simulink model "firmware_requirements_doc_model"  (R2021b)
settings: Solver=VariableStepAuto  StartTime=0.0  StopTime=10.0  RelTol=1e-3
settings Model: Creator=matas  LastModifiedBy=matas

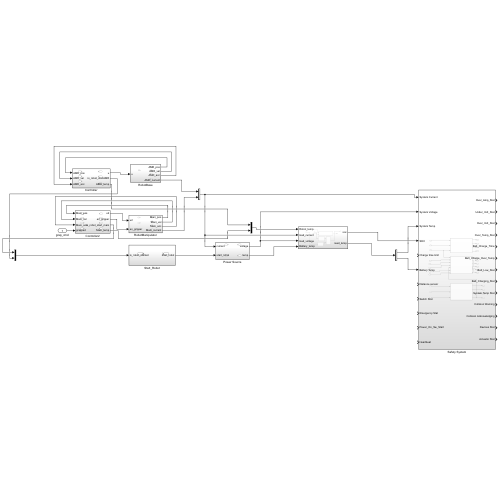
[thumbnail: Simulink's stored preview of the top-level diagram]
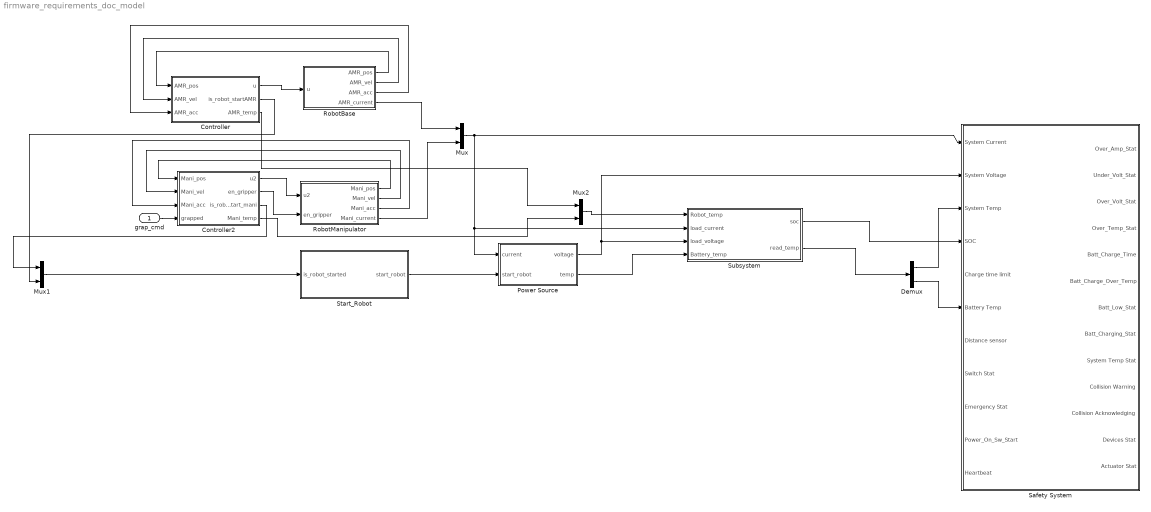
== system firmware_requirements_doc_model ==
  grap_cmd : Inport
  Controller : Subsystem
  Controller2 : Subsystem
  Demux : Demux  Outputs=2
  Mux : Mux  Inputs=2
  Mux1 : Mux  Inputs=2
  Mux2 : Mux  Inputs=2
  Power Source : Subsystem
  RobotBase : Subsystem
  RobotManipulator : Subsystem
  Safety System : Subsystem
  Start_Robot : Subsystem
  Subsystem : Subsystem
  wires:
  Controller2/2(en_gripper) -> RobotManipulator/2(en_gripper)
  Controller2/1(u2) -> RobotManipulator/1(u2)
  Controller/1(u) -> RobotBase/1(u)
  RobotBase/1(AMR_pos) -> Controller/1(AMR_pos)
  RobotBase/2(AMR_vel) -> Controller/2(AMR_vel)
  RobotBase/3(AMR_acc) -> Controller/3(AMR_acc)
  RobotManipulator/1(Mani_pos) -> Controller2/1(Mani_pos)
  RobotManipulator/2(Mani_vel) -> Controller2/2(Mani_vel)
  RobotManipulator/3(Mani_acc) -> Controller2/3(Mani_acc)
  grap_cmd/1 -> Controller2/4(grapped)
  Mux/1 -> Power Source/1(current), Subsystem/2(load_current), Safety System/1(System Current)
  Power Source/1(voltage) -> Subsystem/3(load_voltage), Safety System/2(System Voltage)
  RobotManipulator/4(Mani_current) -> Mux/2
  RobotBase/4(AMR_current) -> Mux/1
  Start_Robot/1(start_robot) -> Power Source/2(start_robot)
  Mux1/1 -> Start_Robot/1(is_robot_started)
  Controller/2(is_robot_startAMR) -> Mux1/2
  Controller2/3(is_robot_start_mani) -> Mux1/1
  Controller/3(AMR_temp) -> Mux2/1
  Controller2/4(Mani_temp) -> Mux2/2
  Demux/1 -> Safety System/3(System Temp)
  Demux/2 -> Safety System/6(Battery Temp)
  Mux2/1 -> Subsystem/1(Robot_temp)
  Power Source/2(temp) -> Subsystem/4(Battery_temp)
  Subsystem/1(soc) -> Safety System/4(SOC)
  Subsystem/2(read_temp) -> Demux/1

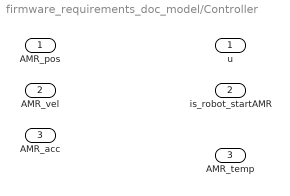
== system firmware_requirements_doc_model/Controller ==
  AMR_pos : Inport
  AMR_vel : Inport  Port=2
  AMR_acc : Inport  Port=3
  u : Outport
  is_robot_startAMR : Outport  Port=2
  AMR_temp : Outport  Port=3

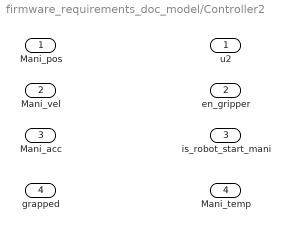
== system firmware_requirements_doc_model/Controller2 ==
  Mani_pos : Inport
  Mani_vel : Inport  Port=2
  Mani_acc : Inport  Port=3
  grapped : Inport  Port=4
  u2 : Outport
  en_gripper : Outport  Port=2
  is_robot_start_mani : Outport  Port=3
  Mani_temp : Outport  Port=4

== system firmware_requirements_doc_model/Power Source ==
  current : Inport
  start_robot : Inport  Port=2
  voltage : Outport
  temp : Outport  Port=2

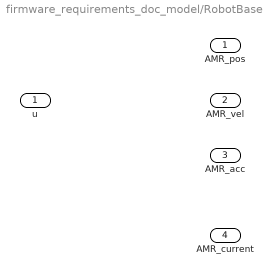
== system firmware_requirements_doc_model/RobotBase ==
  u : Inport
  AMR_pos : Outport
  AMR_vel : Outport  Port=2
  AMR_acc : Outport  Port=3
  AMR_current : Outport  Port=4

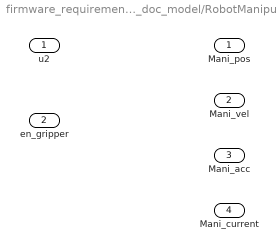
== system firmware_requirements_doc_model/RobotManipulator ==
  u2 : Inport
  en_gripper : Inport  Port=2
  Mani_pos : Outport
  Mani_vel : Outport  Port=2
  Mani_acc : Outport  Port=3
  Mani_current : Outport  Port=4

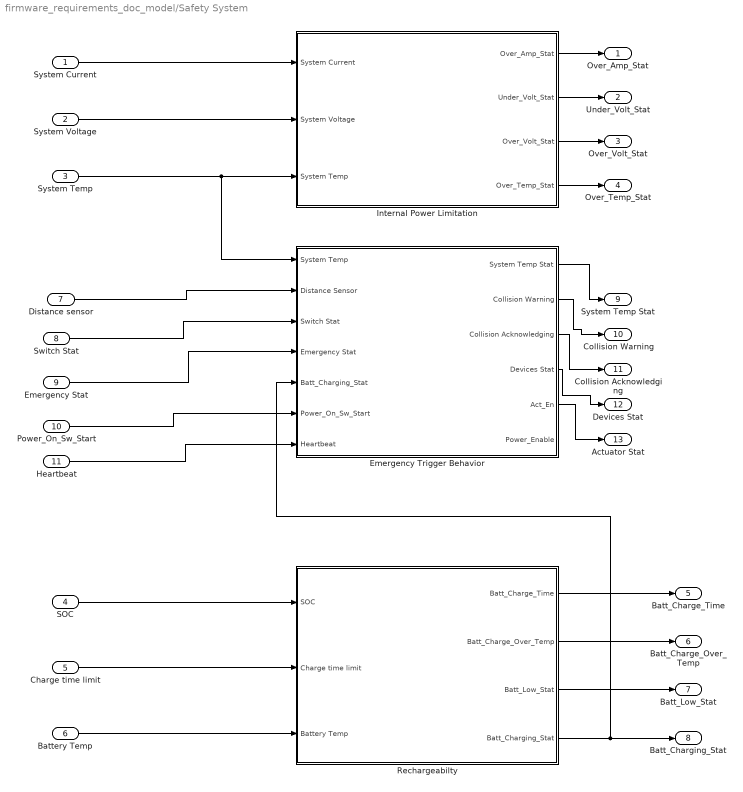
== system firmware_requirements_doc_model/Safety System ==
  System Current : Inport
  System Voltage : Inport  Port=2
  System Temp : Inport  Port=3
  SOC : Inport  Port=4
  Charge time limit : Inport  Port=5
  Battery Temp : Inport  Port=6
  Distance sensor : Inport  Port=7
  Switch Stat : Inport  Port=8
  Emergency Stat : Inport  Port=9
  Power_On_Sw_Start : Inport  Port=10
  Heartbeat : Inport  Port=11
  Emergency Trigger Behavior : Subsystem
  Internal Power Limitation : Subsystem
  Rechargeabilty : Subsystem
  Over_Amp_Stat : Outport
  Under_Volt_Stat : Outport  Port=2
  Over_Volt_Stat : Outport  Port=3
  Over_Temp_Stat : Outport  Port=4
  Batt_Charge_Time : Outport  Port=5
  Batt_Charge_Over_Temp : Outport  Port=6
  Batt_Low_Stat : Outport  Port=7
  Batt_Charging_Stat : Outport  Port=8
  System Temp Stat : Outport  Port=9
  Collision Warning : Outport  Port=10
  Collision Acknowledging : Outport  Port=11
  Devices Stat : Outport  Port=12
  Actuator Stat : Outport  Port=13
  wires:
  System Temp/1 -> Internal Power Limitation/3(System Temp), Emergency Trigger Behavior/1(System Temp)
  System Voltage/1 -> Internal Power Limitation/2(System Voltage)
  Rechargeabilty/1(Batt_Charge_Time) -> Batt_Charge_Time/1
  Rechargeabilty/2(Batt_Charge_Over_Temp) -> Batt_Charge_Over_Temp/1
  Rechargeabilty/3(Batt_Low_Stat) -> Batt_Low_Stat/1
  System Current/1 -> Internal Power Limitation/1(System Current)
  Internal Power Limitation/4(Over_Temp_Stat) -> Over_Temp_Stat/1
  Rechargeabilty/4(Batt_Charging_Stat) -> Emergency Trigger Behavior/5(Batt_Charging_Stat), Batt_Charging_Stat/1
  Internal Power Limitation/1(Over_Amp_Stat) -> Over_Amp_Stat/1
  Internal Power Limitation/2(Under_Volt_Stat) -> Under_Volt_Stat/1
  Internal Power Limitation/3(Over_Volt_Stat) -> Over_Volt_Stat/1
  SOC/1 -> Rechargeabilty/1(SOC)
  Battery Temp/1 -> Rechargeabilty/3(Battery Temp)
  Charge time limit/1 -> Rechargeabilty/2(Charge time limit)
  Distance sensor/1 -> Emergency Trigger Behavior/2(Distance Sensor)
  Emergency Trigger Behavior/4(Devices Stat) -> Devices Stat/1
  Emergency Trigger Behavior/3(Collision Acknowledging) -> Collision Acknowledging/1
  Emergency Trigger Behavior/1(System Temp Stat) -> System Temp Stat/1
  Emergency Trigger Behavior/5(Act_En) -> Actuator Stat/1
  Emergency Trigger Behavior/2(Collision Warning) -> Collision Warning/1
  Switch Stat/1 -> Emergency Trigger Behavior/3(Switch Stat)
  Emergency Stat/1 -> Emergency Trigger Behavior/4(Emergency Stat)
  Power_On_Sw_Start/1 -> Emergency Trigger Behavior/6(Power_On_Sw_Start)
  Heartbeat/1 -> Emergency Trigger Behavior/7(Heartbeat)

== system firmware_requirements_doc_model/Start_Robot ==
  is_robot_started : Inport
  start_robot : Outport

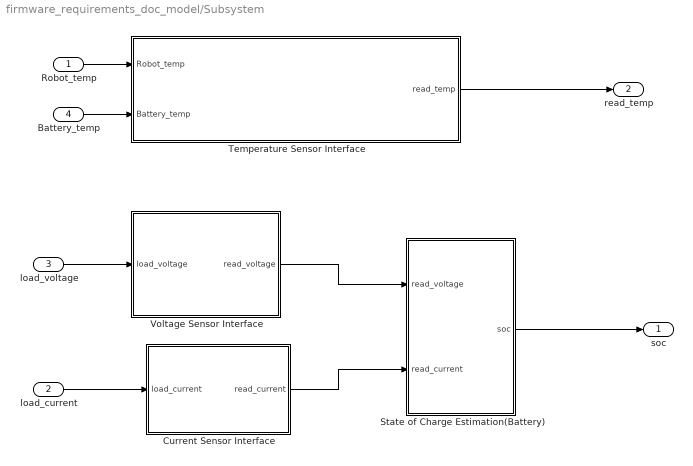
== system firmware_requirements_doc_model/Subsystem ==
  Robot_temp : Inport
  load_current : Inport  Port=2
  load_voltage : Inport  Port=3
  Battery_temp : Inport  Port=4
  Current Sensor Interface : Subsystem
  State of Charge Estimation(Battery) : Subsystem
  Temperature Sensor Interface : Subsystem
  Voltage Sensor Interface : Subsystem
  soc : Outport
  read_temp : Outport  Port=2
  wires:
  Temperature Sensor Interface/1(read_temp) -> read_temp/1
  State of Charge Estimation(Battery)/1(soc) -> soc/1
  Current Sensor Interface/1(read_current) -> State of Charge Estimation(Battery)/2(read_current)
  load_voltage/1 -> Voltage Sensor Interface/1(load_voltage)
  Voltage Sensor Interface/1(read_voltage) -> State of Charge Estimation(Battery)/1(read_voltage)
  Robot_temp/1 -> Temperature Sensor Interface/1(Robot_temp)
  load_current/1 -> Current Sensor Interface/1(load_current)
  Battery_temp/1 -> Temperature Sensor Interface/2(Battery_temp)

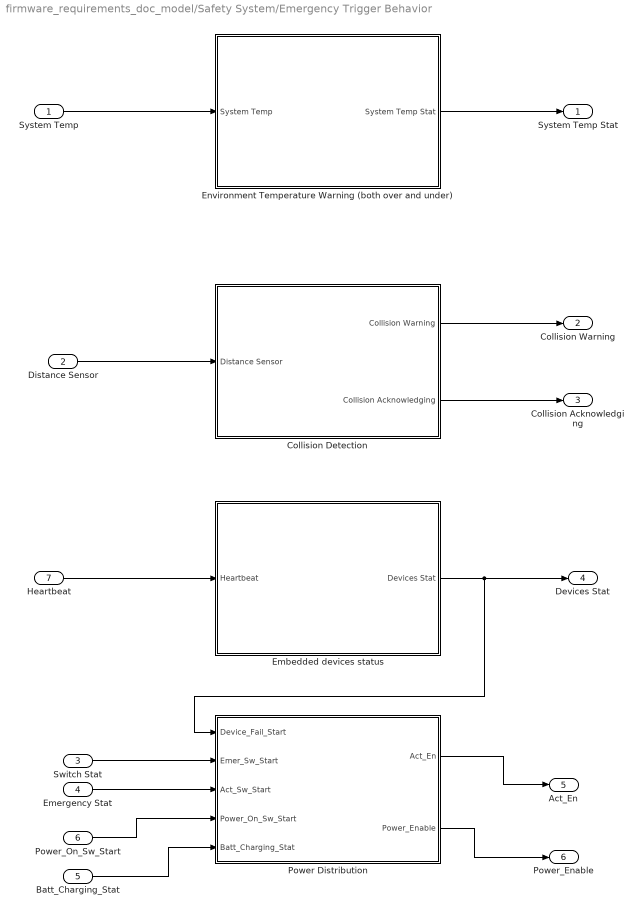
== system firmware_requirements_doc_model/Safety System/Emergency Trigger Behavior ==
  System Temp : Inport
  Distance Sensor : Inport  Port=2
  Switch Stat : Inport  Port=3
  Emergency Stat : Inport  Port=4
  Batt_Charging_Stat : Inport  Port=5
  Power_On_Sw_Start : Inport  Port=6
  Heartbeat : Inport  Port=7
  Collision Detection : Subsystem
  Embedded devices status : Subsystem
  Environment Temperature Warning (both over and under) : Subsystem
  Power Distribution : Subsystem
  System Temp Stat : Outport
  Collision Warning : Outport  Port=2
  Collision Acknowledging : Outport  Port=3
  Devices Stat : Outport  Port=4
  Act_En : Outport  Port=5
  Power_Enable : Outport  Port=6
  wires:
  System Temp/1 -> Environment Temperature Warning (both over and under)/1(System Temp)
  Environment Temperature Warning (both over and under)/1(System Temp Stat) -> System Temp Stat/1
  Distance Sensor/1 -> Collision Detection/1(Distance Sensor)
  Collision Detection/1(Collision Warning) -> Collision Warning/1
  Collision Detection/2(Collision Acknowledging) -> Collision Acknowledging/1
  Power Distribution/1(Act_En) -> Act_En/1
  Switch Stat/1 -> Power Distribution/2(Emer_Sw_Start)
  Emergency Stat/1 -> Power Distribution/3(Act_Sw_Start)
  Batt_Charging_Stat/1 -> Power Distribution/5(Batt_Charging_Stat)
  Power_On_Sw_Start/1 -> Power Distribution/4(Power_On_Sw_Start)
  Embedded devices status/1(Devices Stat) -> Power Distribution/1(Device_Fail_Start), Devices Stat/1
  Power Distribution/2(Power_Enable) -> Power_Enable/1
  Heartbeat/1 -> Embedded devices status/1(Heartbeat)

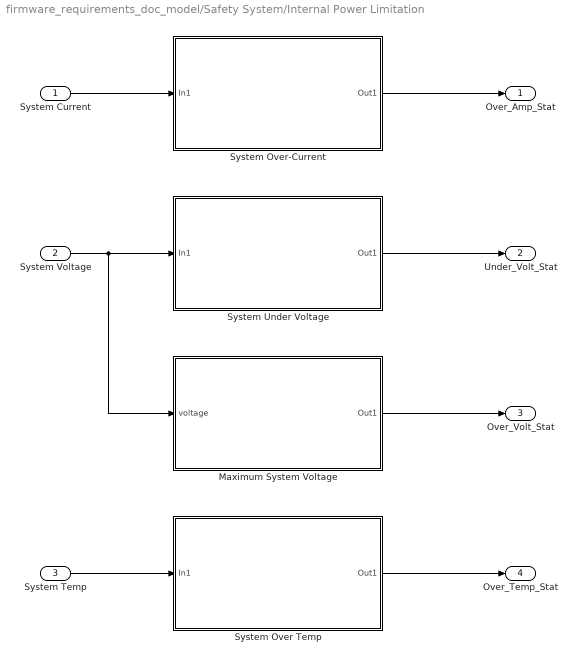
== system firmware_requirements_doc_model/Safety System/Internal Power Limitation ==
  System Current : Inport
  System Voltage : Inport  Port=2
  System Temp : Inport  Port=3
  Maximum System Voltage : Subsystem
  System Over Temp : Subsystem
  System Over-Current : Subsystem
  System Under Voltage : Subsystem
  Over_Amp_Stat : Outport
  Under_Volt_Stat : Outport  Port=2
  Over_Volt_Stat : Outport  Port=3
  Over_Temp_Stat : Outport  Port=4
  wires:
  System Current/1 -> System Over-Current/1(In1)
  System Temp/1 -> System Over Temp/1(In1)
  System Voltage/1 -> Maximum System Voltage/1(voltage), System Under Voltage/1(In1)
  System Over-Current/1(Out1) -> Over_Amp_Stat/1
  System Under Voltage/1(Out1) -> Under_Volt_Stat/1
  Maximum System Voltage/1(Out1) -> Over_Volt_Stat/1
  System Over Temp/1(Out1) -> Over_Temp_Stat/1

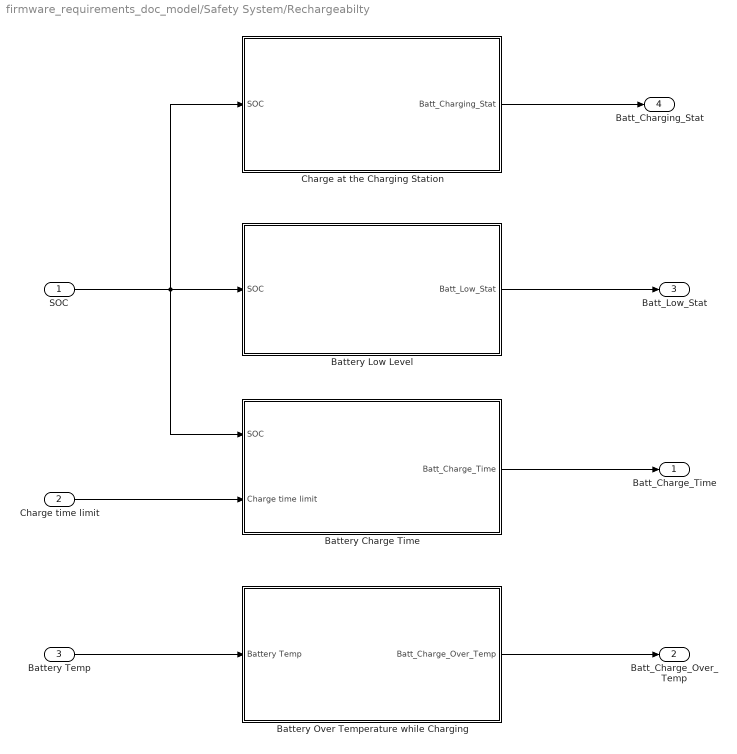
== system firmware_requirements_doc_model/Safety System/Rechargeabilty ==
  SOC : Inport
  Charge time limit : Inport  Port=2
  Battery Temp : Inport  Port=3
  Battery Charge Time : Subsystem
  "Battery Low Level " : Subsystem
  Battery Over Temperature while Charging : Subsystem
  Charge at the Charging Station : Subsystem
  Batt_Charge_Time : Outport
  Batt_Charge_Over_Temp : Outport  Port=2
  Batt_Low_Stat : Outport  Port=3
  Batt_Charging_Stat : Outport  Port=4
  wires:
  Battery Charge Time/1(Batt_Charge_Time) -> Batt_Charge_Time/1
  Charge time limit/1 -> Battery Charge Time/2(Charge time limit)
  Battery Temp/1 -> Battery Over Temperature while Charging/1(Battery Temp)
  Battery Over Temperature while Charging/1(Batt_Charge_Over_Temp) -> Batt_Charge_Over_Temp/1
  "Battery Low Level "/1(Batt_Low_Stat) -> Batt_Low_Stat/1
  SOC/1 -> Battery Charge Time/1(SOC), Charge at the Charging Station/1(SOC), "Battery Low Level "/1(SOC)
  Charge at the Charging Station/1(Batt_Charging_Stat) -> Batt_Charging_Stat/1

== system firmware_requirements_doc_model/Subsystem/Current Sensor Interface ==
  load_current : Inport
  read_current : Outport

== system firmware_requirements_doc_model/Subsystem/State of Charge Estimation(Battery) ==
  read_voltage : Inport
  read_current : Inport  Port=2
  soc : Outport

== system firmware_requirements_doc_model/Subsystem/Temperature Sensor Interface ==
  Robot_temp : Inport
  Battery_temp : Inport  Port=2
  read_temp : Outport

== system firmware_requirements_doc_model/Subsystem/Voltage Sensor Interface ==
  load_voltage : Inport
  read_voltage : Outport

== system firmware_requirements_doc_model/Safety System/Emergency Trigger Behavior/Collision Detection ==
  Distance Sensor : Inport
  Collision Warning : Outport
  Collision Acknowledging : Outport  Port=2

== system firmware_requirements_doc_model/Safety System/Emergency Trigger Behavior/Embedded devices status ==
  Heartbeat : Inport
  Devices Stat : Outport
  wires:
  Heartbeat/1 -> Devices Stat/1

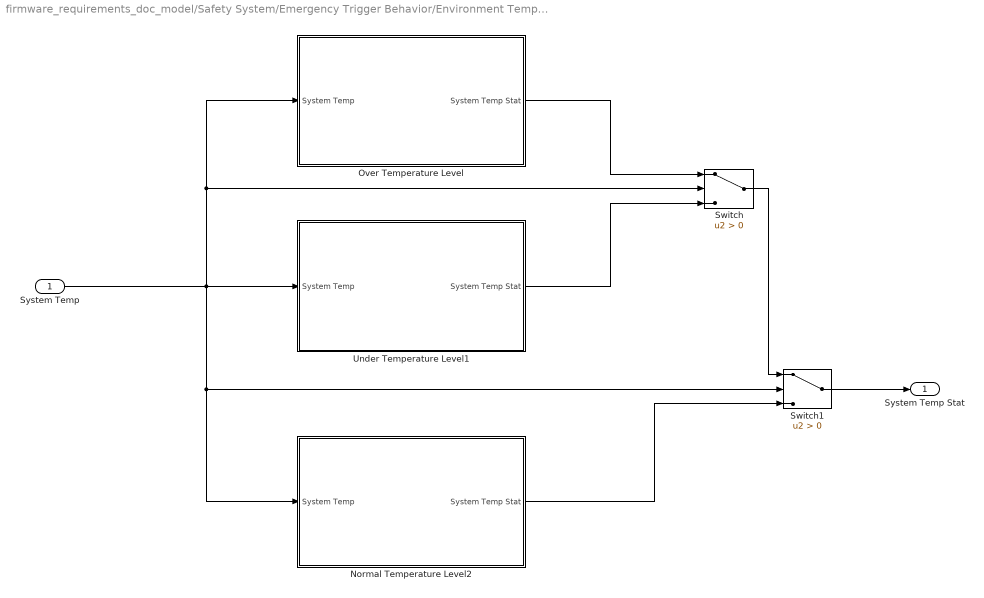
== system firmware_requirements_doc_model/Safety System/Emergency Trigger Behavior/Environment Temperature Warning (both over and under) ==
  System Temp : Inport
  Normal Temperature Level2 : Subsystem
  Over Temperature Level : Subsystem
  Switch : Switch  Criteria=u2 > Threshold
  Switch1 : Switch  Criteria=u2 > Threshold
  Under Temperature Level1 : Subsystem
  System Temp Stat : Outport
  wires:
  System Temp/1 -> Normal Temperature Level2/1(System Temp), Switch1/2, Under Temperature Level1/1(System Temp), Switch/2, Over Temperature Level/1(System Temp)
  Over Temperature Level/1(System Temp Stat) -> Switch/1
  Under Temperature Level1/1(System Temp Stat) -> Switch/3
  Normal Temperature Level2/1(System Temp Stat) -> Switch1/3
  Switch/1 -> Switch1/1
  Switch1/1 -> System Temp Stat/1

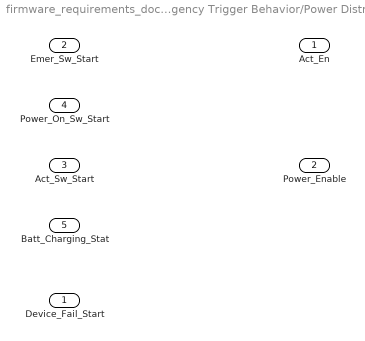
== system firmware_requirements_doc_model/Safety System/Emergency Trigger Behavior/Power Distribution ==
  Device_Fail_Start : Inport
  Emer_Sw_Start : Inport  Port=2
  Act_Sw_Start : Inport  Port=3
  Power_On_Sw_Start : Inport  Port=4
  Batt_Charging_Stat : Inport  Port=5
  Act_En : Outport
  Power_Enable : Outport  Port=2

== system firmware_requirements_doc_model/Safety System/Internal Power Limitation/Maximum System Voltage ==
  voltage : Inport
  Out1 : Outport
  wires:
  voltage/1 -> Out1/1

== system firmware_requirements_doc_model/Safety System/Internal Power Limitation/System Over Temp ==
  In1 : Inport
  Out1 : Outport
  wires:
  In1/1 -> Out1/1

== system firmware_requirements_doc_model/Safety System/Internal Power Limitation/System Over-Current ==
  In1 : Inport
  Out1 : Outport
  wires:
  In1/1 -> Out1/1

== system firmware_requirements_doc_model/Safety System/Internal Power Limitation/System Under Voltage ==
  In1 : Inport
  Out1 : Outport
  wires:
  In1/1 -> Out1/1

== system firmware_requirements_doc_model/Safety System/Rechargeabilty/Battery Charge Time ==
  SOC : Inport
  Charge time limit : Inport  Port=2
  Batt_Charge_Time : Outport
  wires:
  SOC/1 -> Batt_Charge_Time/1

== system firmware_requirements_doc_model/Safety System/Rechargeabilty/Battery Low Level  ==
  SOC : Inport
  Batt_Low_Stat : Outport
  wires:
  SOC/1 -> Batt_Low_Stat/1

== system firmware_requirements_doc_model/Safety System/Rechargeabilty/Battery Over Temperature while Charging ==
  Battery Temp : Inport
  Batt_Charge_Over_Temp : Outport
  wires:
  Battery Temp/1 -> Batt_Charge_Over_Temp/1

== system firmware_requirements_doc_model/Safety System/Rechargeabilty/Charge at the Charging Station ==
  SOC : Inport
  Start to Charge at the Charging Station (Batt_Charging_Stat) : Subsystem
  "Stop to Charge at the Charging Station " : Subsystem
  Switch : Switch  Criteria=u2 > Threshold
  Batt_Charging_Stat : Outport
  wires:
  SOC/1 -> "Stop to Charge at the Charging Station "/1(SOC), Switch/2, Start to Charge at the Charging Station (Batt_Charging_Stat)/1(SOC)
  Switch/1 -> Batt_Charging_Stat/1
  "Stop to Charge at the Charging Station "/1(Batt_Charging_Stat) -> Switch/1
  Start to Charge at the Charging Station (Batt_Charging_Stat)/1(Out1) -> Switch/3

== system firmware_requirements_doc_model/Safety System/Emergency Trigger Behavior/Environment Temperature Warning (both over and under)/Normal Temperature Level2 ==
  System Temp : Inport
  System Temp Stat : Outport
  wires:
  System Temp/1 -> System Temp Stat/1

== system firmware_requirements_doc_model/Safety System/Emergency Trigger Behavior/Environment Temperature Warning (both over and under)/Over Temperature Level ==
  System Temp : Inport
  System Temp Stat : Outport
  wires:
  System Temp/1 -> System Temp Stat/1

== system firmware_requirements_doc_model/Safety System/Emergency Trigger Behavior/Environment Temperature Warning (both over and under)/Under Temperature Level1 ==
  System Temp : Inport
  System Temp Stat : Outport
  wires:
  System Temp/1 -> System Temp Stat/1

== system firmware_requirements_doc_model/Safety System/Rechargeabilty/Charge at the Charging Station/Start to Charge at the Charging Station (Batt_Charging_Stat) ==
  SOC : Inport
  Out1 : Outport
  wires:
  SOC/1 -> Out1/1

== system firmware_requirements_doc_model/Safety System/Rechargeabilty/Charge at the Charging Station/Stop to Charge at the Charging Station  ==
  SOC : Inport
  Batt_Charging_Stat : Outport
  wires:
  SOC/1 -> Batt_Charging_Stat/1
